simulink subsystem "FT"  (R2022a)
settings: Solver=VariableStepAuto  StartTime=0.0  StopTime=10.0  RelTol=1e-3
values from neighbouring files (symbols this model uses):
  Den = [1 2*ep*wn wn^2]    [principal.m]
  Num = wn^2    (= 16)    [principal.m]
  variancia = var    [simular.m]
settings Model: Creator=jaedson  LastModifiedBy=jaedson

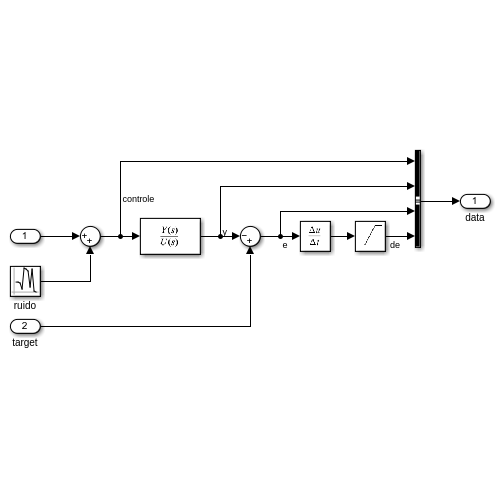
[thumbnail: Simulink's stored preview of the top-level diagram]
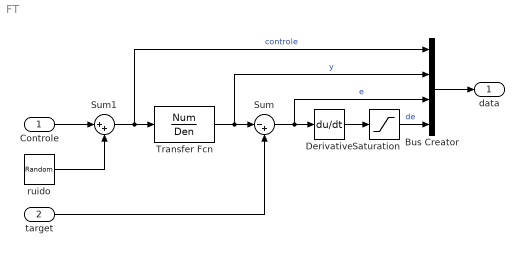
== system FT ==
  Controle : Inport
  target : Inport  Port=2
  Bus Creator : BusCreator  Inputs=4
  Derivative : Derivative
  Saturation : Saturate  UpperLimit=5  LowerLimit=-5  LinearizeAsGain=off  ZeroCross=off
  Sum : Sum  Inputs=|-+
  Sum1 : Sum  Inputs=|++
  Transfer Fcn : TransferFcn  Numerator=Num  Denominator=Den
  ruido : RandomNumber  Variance=variancia  SampleTime=0.001
  data : Outport
  wires:
  Transfer Fcn/1 -> Bus Creator/2, Sum/1  "y"
  Sum/1 -> Derivative/1, Bus Creator/3  "e"
  Sum1/1 -> Bus Creator/1, Transfer Fcn/1  "controle"
  Controle/1 -> Sum1/1
  ruido/1 -> Sum1/2
  Bus Creator/1 -> data/1
  target/1 -> Sum/2
  Derivative/1 -> Saturation/1
  Saturation/1 -> Bus Creator/4  "de"
